simulink model "Z_trajectory_with_only_functions"  (R2018b)
settings: Solver=FixedStepAuto  StartTime=0.0  StopTime=inf  RelTol=1e-3  EnableMultiTasking=on
undefined symbols (not defined in the file or in its folder): dev, Main, pwm_output0
libraries: px4Sensorslib x2, px4lib x1, px4uORBlib x1
settings Model: ExtModeTrigDuration=10  Creator=Tejas Rajopadhye  LastModifiedBy=Tejas Rajopadhye
settings SolverCC: PositivePriorityOrder=on  AutoInsertRateTranBlk=on
settings OptimizationCC: EnhancedBackFolding=on  PassReuseOutputArgsAs=Individual arguments  MaxStackSize=64  OptimizeBlockOrder=speed  DifferentSizesBufferReuse=on  OptimizationCustomize=off
settings DebuggingCC: ParameterTunabilityLossMsg=error
settings HardwareCC: ProdBitPerPointer=32  ProdBitPerSizeT=32  ProdBitPerPtrDiffT=32  ProdLargestAtomicInteger=Long  ProdLargestAtomicFloat=Double  ProdWordSize=32  ProdLongLongMode=on  ProdHWDeviceType=ARM Compatible->ARM Cortex
settings SFSimCC: MATLABDynamicMemAlloc=off
settings RTWCC: SystemTargetFile=ert.tlc  HardwareBoard=PX4 Pixhawk 4  TLCOptions="-aInlineSetEventsForThisBaseRateFcn=TLC_FALSE -aSuppressMultiTaskScheduler=TLC_FALSE  -aRateBasedStepFcn=0"  TemplateMakefile=ert_default_tmf  GenerateReport=on  Toolchain=GNU Tools for PX4 Autopilots  IncludeHyperlinkInReport=on  LaunchReport=on  TargetLang=C++  GenerateTraceInfo=on  GenerateTraceReport=on  GenerateTraceReportSl=on  GenerateTraceReportSf=on  GenerateTraceReportEml=on
settings CodeAppCC: ForceParamTrailComments=on  IgnoreCustomStorageClasses=off  OperatorAnnotations=on  SimulinkDataObjDesc=on  SFDataObjDesc=on  InsertBlockDesc=on

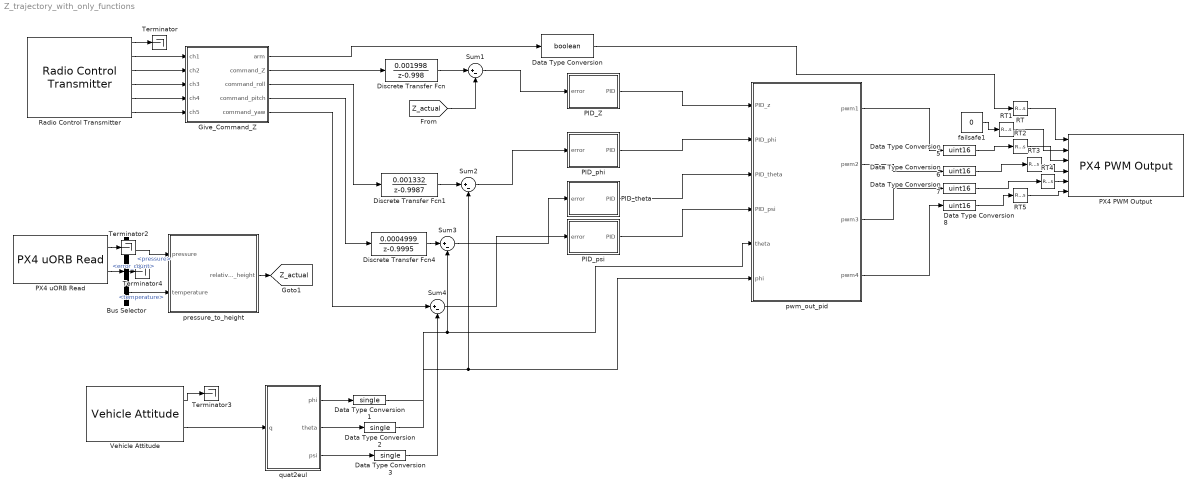
== system Z_trajectory_with_only_functions ==
  Bus Selector : BusSelector  OutputSignals=pressure,error_count,temperature
  Data Type Conversion : DataTypeConversion  OutDataTypeStr=boolean
  Data Type Conversion1 : DataTypeConversion  OutDataTypeStr=single
  Data Type Conversion2 : DataTypeConversion  OutDataTypeStr=single
  Data Type Conversion3 : DataTypeConversion  OutDataTypeStr=single
  Data Type Conversion{5..8} (4 alike) : DataTypeConversion  OutDataTypeStr=uint16
  Discrete Transfer Fcn : DiscreteTransferFcn  Numerator=[0.001998]  Denominator=[1 -0.998]
  Discrete Transfer Fcn1 : DiscreteTransferFcn  Numerator=[0.001332]  Denominator=[1 -0.9987]
  Discrete Transfer Fcn4 : DiscreteTransferFcn  Numerator=[0.0004999]  Denominator=[1 -0.9995]
  Give_Command_Z : MATLAB Function  TreatAsAtomicUnit=on
  PID_Z : MATLAB Function  TreatAsAtomicUnit=on
  PID_phi : MATLAB Function  TreatAsAtomicUnit=on
  PID_psi : MATLAB Function  TreatAsAtomicUnit=on
  PID_theta : MATLAB Function  TreatAsAtomicUnit=on
  PX4 PWM Output : px4lib/PX4 PWM Output  pwmDevice=Main (/dev/pwm_output0)  pwmChannel1_=on  pwmChannel2_=on  pwmChannel3_=on  pwmChannel4_=on  pwmChannel5_=off  pwmChannel6_=off  pwmChannel7_=off  pwmChannel8_=off  forceTerminateFailsafe=off  outputErrorStatus=off
      settings: SourceProductName=Embedded Coder Support Package for PX4 Autopilots  SourceProductBaseCode=PX4AUTOPILOTS
  PX4 uORB Read : px4uORBlib/PX4 uORB Read  uORBTopic=sensor_baro  sampleTime=-1  BlockingMode=off  BlockTimeout=1e-3
      settings: SourceProductName=Embedded Coder Support Package for PX4 Autopilots
  RT{,1..5} (6 alike) : RateTransition  OutPortSampleTime=0.002
  Radio Control Transmitter : px4Sensorslib/Radio Control Transmitter  channel1=on  channel2=on  channel3=on  channel4=on  channel5=on  channel6=off  channel7=off  channel8=off  channel_count=off  rssi=off  rc_input_source=off  timestamp_last_signal=off  time_stamp=off  sampleTime=1/250  BlockingMode=off  BlockTimeout=5
      settings: SourceProductName=Embedded Coder Support Package for PX4 Autopilots
  Sum{1..4} (4 alike) : Sum  Inputs=|+-
  Terminator{,2..4} (4 alike) : Terminator
  Vehicle Attitude : px4Sensorslib/Vehicle Attitude  rollRate=off  pitchRate=off  yawRate=off  quaternion=on  uorbTimeStamp=off  BlockingMode=off  BlockTimeout=0.001  sampleTime=1/250
      settings: SourceProductName=Embedded Coder Support Package for PX4 Autopilots
  failsafe1 : Constant  Value=0  OutDataTypeStr=boolean  SampleTime=0.01
  pressure_to_height : MATLAB Function  TreatAsAtomicUnit=on
  pwm_out_pid : MATLAB Function  TreatAsAtomicUnit=on
  quat2eul : MATLAB Function  TreatAsAtomicUnit=on
  tag scope: Z_actual=global
  wires:
  Radio Control Transmitter/1 -> Terminator/1
  Radio Control Transmitter/2 -> Give_Command_Z/1(ch1)
  Radio Control Transmitter/6 -> Give_Command_Z/5(ch5)
  Give_Command_Z/1(arm) -> Data Type Conversion/1
  failsafe1/1 -> RT1/1
  Data Type Conversion5/1 -> RT2/1
  Data Type Conversion8/1 -> RT5/1
  Data Type Conversion6/1 -> RT3/1
  Data Type Conversion7/1 -> RT4/1
  Vehicle Attitude/1 -> Terminator3/1
  Sum3/1 -> PID_theta/1(error)
  Sum4/1 -> PID_psi/1(error)
  PID_phi/1(PID) -> pwm_out_pid/2(PID_phi)
  PID_theta/1(PID) -> pwm_out_pid/3(PID_theta)
  PID_psi/1(PID) -> pwm_out_pid/4(PID_psi)
  Sum1/1 -> PID_Z/1(error)
  PID_Z/1(PID) -> pwm_out_pid/1(PID_z)
  [Z_actual] -> Sum1/2
  Vehicle Attitude/2 -> quat2eul/1(q)
  quat2eul/3(psi) -> Data Type Conversion3/1
  quat2eul/2(theta) -> Data Type Conversion2/1
  quat2eul/1(phi) -> Data Type Conversion1/1
  Sum2/1 -> PID_phi/1(error)
  PX4 uORB Read/2 -> Bus Selector/1
  PX4 uORB Read/1 -> Terminator2/1
  Bus Selector/2 -> Terminator4/1  "<error_count>"
  Bus Selector/1 -> pressure_to_height/1(pressure)  "<pressure>"
  Bus Selector/3 -> pressure_to_height/2(temperature)  "<temperature>"
  pressure_to_height/1(relative_height) -> [Z_actual]
  Data Type Conversion/1 -> RT/1
  Data Type Conversion1/1 -> pwm_out_pid/6(phi), Sum2/2
  Data Type Conversion2/1 -> pwm_out_pid/5(theta), Sum3/2
  Data Type Conversion3/1 -> Sum4/2
  pwm_out_pid/1(pwm1) -> Data Type Conversion5/1
  pwm_out_pid/2(pwm2) -> Data Type Conversion6/1
  pwm_out_pid/3(pwm3) -> Data Type Conversion7/1
  pwm_out_pid/4(pwm4) -> Data Type Conversion8/1
  RT/1 -> PX4 PWM Output/1
  RT1/1 -> PX4 PWM Output/2
  RT2/1 -> PX4 PWM Output/3
  RT3/1 -> PX4 PWM Output/4
  RT4/1 -> PX4 PWM Output/5
  RT5/1 -> PX4 PWM Output/6
  Give_Command_Z/2(command_Z) -> Discrete Transfer Fcn/1
  Discrete Transfer Fcn/1 -> Sum1/1
  Discrete Transfer Fcn1/1 -> Sum2/1
  Discrete Transfer Fcn4/1 -> Sum3/1
  Give_Command_Z/5(command_yaw) -> Sum4/1
  Radio Control Transmitter/3 -> Give_Command_Z/2(ch2)
  Radio Control Transmitter/4 -> Give_Command_Z/3(ch3)
  Radio Control Transmitter/5 -> Give_Command_Z/4(ch4)
  Give_Command_Z/3(command_roll) -> Discrete Transfer Fcn1/1
  Give_Command_Z/4(command_pitch) -> Discrete Transfer Fcn4/1

== matlab function Z_trajectory_with_only_functions/pwm_out_pid ==
  data: PID_z input; PID_phi input; PID_theta input; PID_psi input; pwm1 output; pwm2 output; pwm3 output; pwm4 output; theta input; phi input
function [pwm1, pwm2, pwm3, pwm4] = MIXER(PID_z, PID_phi, PID_theta, PID_psi ,theta, phi)
Ixx = single(0.047);
Iyy = single(0.047);
Izz = single(0.094);

g = single(9.81);
l = single(0.225);
m = single(0.93);
ct = single(0.0984);    % Values from doc
cm = single(0.00679);   % Values from doc

%Complete the instrutions
T = m*g + PID_z /(cos(theta)*cos(phi)); %U4 This is a more logical way of writing the torque term
tauphi = PID_phi; %*Ixx;
tautheta = PID_theta; %*Iyy;
taupsi = PID_psi; %*Izz;

% w1 w2 .... Made changes in the signs according to our calculations and
% model... make sure you do the right connections on the setup

w1 = T/(4*ct) - tautheta/(2*ct*l) - taupsi/(4*cm);
w2 = T/(4*ct) - tauphi/(2*ct*l) + taupsi/(4*cm);
w3 = T/(4*ct) + tautheta/(2*ct*l) - taupsi/(4*cm);
w4 = T/(4*ct) + tauphi/(2*ct*l) + taupsi/(4*cm);

% taupsi = u3
% tautheta = u2
% tauphi = u1
% T = u4

% Taking sqrt of all omega's
w1 = sqrt(w1);
w2 = sqrt(w2);
w3 = sqrt(w3);
w4 = sqrt(w4);


% convert omegas to Pwm values and give the output to pwm block
% From this answer that i got from net about working of ESC's (https://electronics.stackexchange.com/questions/42616/how-to-use-an-esc)
% 100 % Pwm --> 2.0ms (@50hz) --> maxSpeed (11000rpm)
% Using that logic 2,5ms*Xrpm/ 11000rpm will give us the required PWM

pwm1 = (w1*2.0e-3)/11000;
pwm2 = (w2*2.0e-3)/11000;
pwm3 = (w3*2.0e-3)/11000;
pwm4 = (w4*2.0e-3)/11000;

if (pwm1 < single(900) || pwm2 < single(900) || pwm3 < single(900) || pwm4 < single(900))
    pwm1 = single(900);
    pwm2 = single(900);
    pwm3 = single(900);
    pwm4 = single(900);
end

if (pwm1 > single(1950) || pwm2 > single(1950) || pwm3 < single(1950) || pwm4 < single(1950))
    pwm1 = single(1950);
    pwm2 = single(1950);
    pwm3 = single(1950);
    pwm4 = single(1950);
end

[pwm1, pwm2, pwm3, pwm4];

== matlab function Z_trajectory_with_only_functions/Give_Command_Z ==
  data: arm output; ch1 input; ch2 input; ch3 input; ch4 input; command_Z output; ch5 input; command_roll output; command_pitch output; command_yaw output
function [arm, command_Z, command_roll, command_pitch, command_yaw] = Commands(ch1, ch2, ch3, ch4, ch5)
ch1 = single(ch1);
command_Z =  3; %(ch1 - 1000)/100; %for z trajecctory from 0 to 10m
if (ch5 > single(1500))
    arm = true;
else
    arm = false;
end

== matlab function Z_trajectory_with_only_functions/pressure_to_height ==
  data: pressure input; relative_height output; temperature input
function relative_height = covert_pressure_to_height(pressure, temperature)
R = single(287.058);
g = single(9.81);
temperature = temperature + single(273.15); %convert to kelvin from degrees

persistent itr;
if isempty(itr)
    itr = 0;
end

persistent init_pressure;
if isempty(init_pressure)
    init_pressure = single(944.77);
end

persistent initial_temp;
if isempty(initial_temp)
    initial_temp = temperature;
end

if (itr == 0)
    initial_pressure = pressure;
    itr = itr + 1;
else
    initial_pressure = single(init_pressure);
end

if (isreal(log(initial_pressure/pressure)))
    log_value = log(initial_pressure/pressure);
else
    log_value = 0;
end

init_pressure = single(initial_pressure);

relative_height = single(((R*initial_temp)/g)*log_value);

== matlab function Z_trajectory_with_only_functions/PID_Z ==
  data: error input; PID output
function PID = fcn(error)
Ki = single(2.5);
Kp = single(20.5);
Kd = single(55.5);
persistent error_integral;
persistent previous_error;
if isempty(error_integral)
    error_integral = single(0);
end
if isempty(previous_error)
    previous_error = error;
end
integral_time = single(0.004);

error_integral= error_integral + error*integral_time;
if (error_integral > single(10))
    error_integral = single(10);
end
if (error_integral < single(-10))
    error_integral = single(-10);
end

PID = single(Kp*error + Ki*(error_integral) + Kd*((error - previous_error)/integral_time));
previous_error = error;

== matlab function Z_trajectory_with_only_functions/PID_phi ==
  data: error input; PID output
function PID = fcn(error)
Ki = single(0.001);
Kp = single(30);
Kd = single(13);
persistent error_integral;
persistent previous_error;
if isempty(error_integral)
    error_integral = single(0);
end
if isempty(previous_error)
    previous_error = error;
end
integral_time = single(0.004);

error_integral= error_integral + error*integral_time;


PID = single(Kp*error + Ki*(error_integral) + Kd*((error - previous_error)/integral_time));
previous_error = error;

== matlab function Z_trajectory_with_only_functions/PID_theta ==
  data: error input; PID output
function PID = fcn(error)
Ki = single(0.01);
Kp = single(11.05);
Kd = single(10.05);
persistent error_integral;
persistent previous_error;
if isempty(error_integral)
    error_integral = single(0);
end
if isempty(previous_error)
    previous_error = error;
end
integral_time = single(0.004);

error_integral= error_integral + error*integral_time;


PID = single(Kp*error + Ki*(error_integral) + Kd*((error - previous_error)/integral_time));
previous_error = error;

== matlab function Z_trajectory_with_only_functions/PID_psi ==
  data: error input; PID output
function PID = fcn(error)
Ki = single(2);
Kp = single(100);
Kd = single(1);
persistent error_integral;
persistent previous_error;
if isempty(error_integral)
    error_integral = single(0);
end
if isempty(previous_error)
    previous_error = error;
end
integral_time = single(0.004);

error_integral= error_integral + error*integral_time;

PID = single(Kp*error + Ki*(error_integral) + Kd*((error - previous_error)/integral_time));
previous_error = error;

== matlab function Z_trajectory_with_only_functions/quat2eul ==
  data: q input; phi output; theta output; psi output
function [phi,theta,psi] = quat2eul(q)
% Conversion from Quaternion to Euler angles based on the PX4 Firmware
% v1.6.5 release.
% 
% Quaternion -> DCM -> Euler Angles
% INPUT:
%   q: Quaternion vector of the format: (a + bi + cj + dk)
% OUTPUT:
%   [phi,theta,psi]: Euler angles in radians.
% 
 
    a = q(1);
    b = q(2);
    c = q(3);
    d = q(4);

    aSq = a*a;
    bSq = b*b;
    cSq = c*c;
    dSq = d*d;

    d_pi2 = pi/2;

    % quaternion_to_dcm
    dcm00 = aSq + bSq - cSq - dSq;
    % dcm01 = 2*(b*c - a*d);
    dcm02 = 2*(a*c + b*d);
    dcm10 = 2*(b*c + a*d);
    % dcm11 = aSq - bSq + cSq - dSq;
    dcm12 = 2*(c*d - a*b);
    dcm20 = 2*(b*d - a*c);
    dcm21 = 2*(a*b + c*d);
    dcm22 = aSq - bSq - cSq + dSq;

    % dcm_to_euler
    theta = asin(-dcm20);
    if abs(theta - d_pi2) < 1.0e-3
        phi = single(0.0);
        psi = atan2(dcm12, dcm02);
    elseif abs(theta + d_pi2) < 1.0e-3
        phi = single(0.0);
        psi = atan2(-dcm12, -dcm02);
    else
        phi = atan2(dcm21, dcm22);
        psi = atan2(dcm10, dcm00);
    end

end
